simulink model "Simscape_CAD_Raibert"  (R2022a)
settings: Solver=VariableStepAuto  StartTime=0.0  StopTime=6  FixedStep=1E-6  MaxStep=1E-5  RelTol=1E-9
undefined symbols (not defined in the file or in its folder): arm_l, arm_r, arm_spacing, base_h, base_r, contactTime, desired_speed, height_plane, hip_bend_factor, hip_fuzz, initHip, initKnee, k_landing_angle, knee_bend_factor, knee_fuzz, lower_leg_length, max_torque, plane_x, plane_y, plane_z, upper_leg_length, X, Y, Z
libraries: sm_lib x46, nesl_utility x14, slpidlib x6, simulink x1
(part 1 of 3)
settings Model: SimulationMode=accelerator  Creator=Bradley Kwan  LastModifiedBy=jack3
settings SolverCC: ZeroCrossAlgorithm=Adaptive  AlgebraicLoopSolver=TrustRegion
settings DebuggingCC: UnconnectedInputMsg=warning  UnconnectedOutputMsg=warning  UnconnectedLineMsg=warning  SFMachineParentedDataDiag=warning
settings RTWCC: DLArmComputeVersion=19.05
settings ExplorerConfigSet: InternalSimMechanicsExplorerSettings="<ExplorerConfiguration><canonicalview>default</canonicalview><AnimationSetting><BasePlaybackSpeed>1.0</BasePlaybackSpeed><PlaybackSpeedFactor>1.0</PlaybackSpeedFactor></AnimationSetting><TilePanel><TileInfo><Tiles Columns=\"1\" Count=\"1\" Rows=\"1\"><Column Weight=\"1\"/><Row Weight=\"1\"/><Tile Height=\"1\" Width=\"1\" X=\"0\" Y=\"0\"/></Tiles></TileInfo><SceneInfo><SceneViewer><BGColor><R>0.60000002384185791</R><G>0.60000002384185791</G><B>0.60000002384185791</B></BGColor><Camera><DoPerspective>off</DoPerspective><Position><X>1.00328009491088266</X><Y>0.290256330840329813</Y><Z>0.225430262208942023</Z></Position><Center><X>0.0386568878869436583</X><Y>0.0720479721949161545</Y><Z>0.0774870951204086611</Z></Center><Up><X>-0.177845876958520221</X><Y>0.124361864790182741</Y><Z>0.976168515490416722</Z></Up><ViewLimDist>1</ViewLimDist><YLim>0.220252111002240375</YLim><XLim>0.209173030971946589</XLim></Camera></SceneViewer></SceneInfo></TilePanel><MechEditorPanel><Cameras/><GfxPanelCameraMap/><VideoCreator><PlaybackSpeedRatio>1.0</PlaybackSpeedRatio><FrameRate>60</FrameRate><VideoFormat>MPEG-4</VideoFormat><FrameSize>auto</FrameSize></VideoCreator></MechEditorPanel></ExplorerConfiguration>"

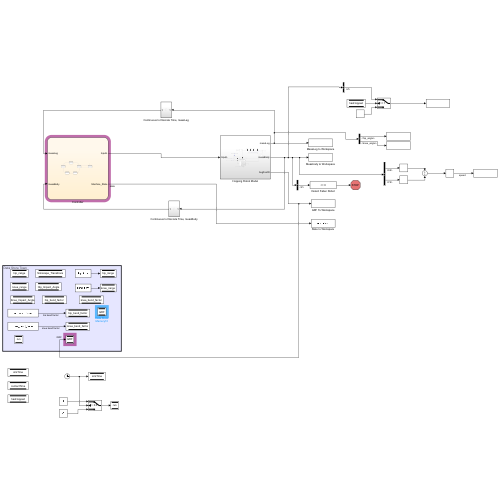
[thumbnail: Simulink's stored preview of the top-level diagram]
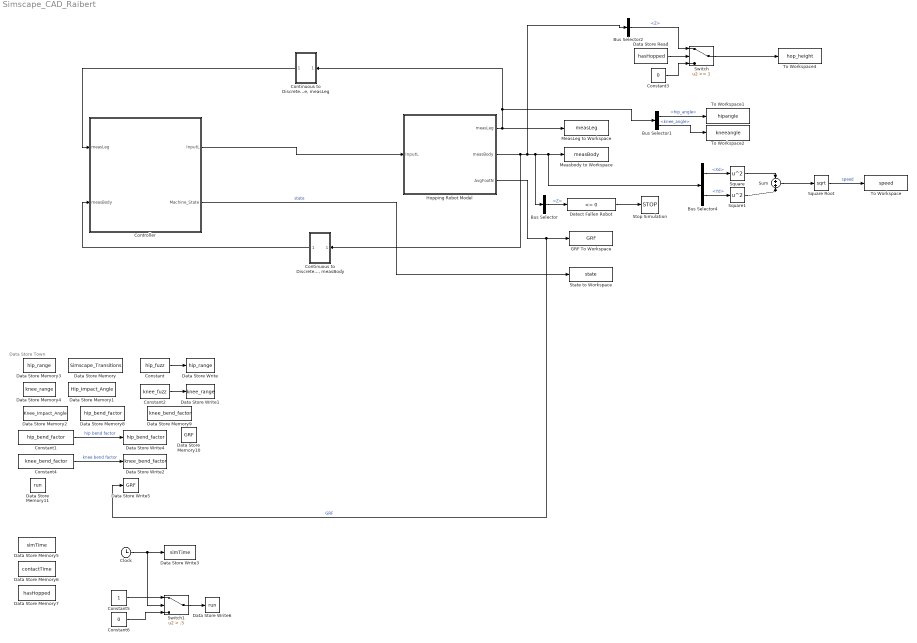
== system Simscape_CAD_Raibert ==
  note: Data Store Town
  Bus Selector : BusSelector  OutputSignals=Z
  Bus Selector1 : BusSelector  OutputSignals=hip_angle,knee_angle
  Bus Selector2 : BusSelector  OutputSignals=Z
  Bus Selector4 : BusSelector  OutputSignals=Xd,Yd
  Clock : Clock
  Constant : Constant  Value=hip_fuzz
  Constant1 : Constant  Value=hip_bend_factor
  Constant2 : Constant  Value=knee_fuzz
  Constant3 : Constant  Value=0
  Constant4 : Constant  Value=knee_bend_factor
  Constant5 : Constant
  Constant6 : Constant  Value=0
  "Continuous to Discrete Time, measBody" : Subsystem
  "Continuous to Discrete Time, measLeg" : Subsystem
  Controller : Stateflow chart  TreatAsAtomicUnit=on
  Data Store Memory : DataStoreMemory  DataStoreName=Simscape_Transitions  WriteAfterWriteMsg=warning  ShowAdditionalParam=off  OutDataTypeStr=double  Dimensions=3
  Data Store Memory1 : DataStoreMemory  DataStoreName=Hip_Impact_Angle  WriteAfterWriteMsg=warning  ShowAdditionalParam=off  OutDataTypeStr=double
  Data Store Memory10 : DataStoreMemory  DataStoreName=GRF  WriteAfterWriteMsg=warning  ShowAdditionalParam=off  OutDataTypeStr=double
  Data Store Memory11 : DataStoreMemory  DataStoreName=run  WriteAfterWriteMsg=warning  ShowAdditionalParam=off  OutDataTypeStr=double
  Data Store Memory2 : DataStoreMemory  DataStoreName=Knee_Impact_Angle  WriteAfterWriteMsg=warning  ShowAdditionalParam=off  OutDataTypeStr=double
  Data Store Memory3 : DataStoreMemory  DataStoreName=hip_range  WriteAfterWriteMsg=warning  ShowAdditionalParam=off  OutDataTypeStr=double
  Data Store Memory4 : DataStoreMemory  DataStoreName=knee_range  WriteAfterWriteMsg=warning  ShowAdditionalParam=off  OutDataTypeStr=double
  Data Store Memory5 : DataStoreMemory  DataStoreName=simTime  WriteAfterWriteMsg=warning  ShowAdditionalParam=off  OutDataTypeStr=double
  Data Store Memory6 : DataStoreMemory  DataStoreName=contactTime  WriteAfterWriteMsg=warning  ShowAdditionalParam=off  OutDataTypeStr=double
  Data Store Memory7 : DataStoreMemory  DataStoreName=hasHopped  WriteAfterWriteMsg=warning  ShowAdditionalParam=off  OutDataTypeStr=double
  Data Store Memory8 : DataStoreMemory  DataStoreName=hip_bend_factor  WriteAfterWriteMsg=warning  ShowAdditionalParam=off  OutDataTypeStr=double
  Data Store Memory9 : DataStoreMemory  DataStoreName=knee_bend_factor  WriteAfterWriteMsg=warning  ShowAdditionalParam=off  OutDataTypeStr=double
  Data Store Read : DataStoreRead  DataStoreName=hasHopped  IndexOptions=Index vector (dialog)  Indices=1  OutputSizes=1
  Data Store Write : DataStoreWrite  DataStoreName=hip_range  IndexOptions=Index vector (dialog)  Indices=1  OutputSizes=1
  Data Store Write1 : DataStoreWrite  DataStoreName=knee_range  IndexOptions=Index vector (dialog)  Indices=1  OutputSizes=1
  Data Store Write2 : DataStoreWrite  DataStoreName=knee_bend_factor  IndexOptions=Index vector (dialog)  Indices=1  OutputSizes=1
  Data Store Write3 : DataStoreWrite  DataStoreName=simTime  IndexOptions=Index vector (dialog)  Indices=1  OutputSizes=1
  Data Store Write4 : DataStoreWrite  DataStoreName=hip_bend_factor  IndexOptions=Index vector (dialog)  Indices=1  OutputSizes=1
  Data Store Write5 : DataStoreWrite  DataStoreName=GRF  IndexOptions=Index vector (dialog)  Indices=1  OutputSizes=1
  Data Store Write6 : DataStoreWrite  DataStoreName=run  IndexOptions=Index vector (dialog)  Indices=1  OutputSizes=1
  Detect Fallen Robot : simulink/Logic and Bit Operations/Compare To Constant  relop=<=  const=0  OutDataTypeStr=boolean
  GRF To Workspace : ToWorkspace  VariableName=GRF  SampleTime=-1
  Hopping Robot Model : Subsystem
  MeasLeg to Workspace : ToWorkspace  VariableName=measLeg  SampleTime=-1
  Measbody to Workspace : ToWorkspace  VariableName=measBody  SampleTime=-1
  Square : Math  Operator=square
  Square Root : Sqrt
  Square1 : Math  Operator=square
  State to Workspace : ToWorkspace  VariableName=state  SampleTime=-1
  Stop Simulation : Stop
  Sum : Sum  Inputs=+|+
  Switch : Switch  Threshold=1  SaturateOnIntegerOverflow=off  InputSameDT=off
  Switch1 : Switch  Criteria=u2 > Threshold  Threshold=.5  SaturateOnIntegerOverflow=off  InputSameDT=off
  To Workspace : ToWorkspace  VariableName=speed  SaveFormat=Timeseries  SampleTime=-1
  To Workspace1 : ToWorkspace  VariableName=hipangle  SaveFormat=Timeseries  SampleTime=-1
  To Workspace2 : ToWorkspace  VariableName=kneeangle  SaveFormat=Timeseries  SampleTime=-1
  To Workspace4 : ToWorkspace  VariableName=hop_height  SaveFormat=Timeseries  SampleTime=-1
  wires:
  Hopping Robot Model/2(measBody) -> "Continuous to Discrete Time, measBody"/1(In1), Bus Selector2/1, Bus Selector/1, Bus Selector4/1, Measbody to Workspace/1
  Bus Selector/1 -> Detect Fallen Robot/1  "<Z>"
  Detect Fallen Robot/1 -> Stop Simulation/1
  Hopping Robot Model/3(AvgFootN) -> Data Store Write5/1, GRF To Workspace/1  "GRF"
  Controller/1(InputL) -> Hopping Robot Model/1(InputL)
  Constant1/1 -> Data Store Write4/1  "hip bend factor"
  Controller/2(Machine_State) -> State to Workspace/1  "state"
  Constant4/1 -> Data Store Write2/1  "knee bend factor"
  Constant/1 -> Data Store Write/1
  Constant2/1 -> Data Store Write1/1
  Bus Selector4/2 -> Square1/1  "<Yd>"
  Bus Selector4/1 -> Square/1  "<Xd>"
  Square/1 -> Sum/1
  Square1/1 -> Sum/2
  Sum/1 -> Square Root/1
  Square Root/1 -> To Workspace/1  "speed"
  "Continuous to Discrete Time, measBody"/1(Out1) -> Controller/2(measBody)
  "Continuous to Discrete Time, measLeg"/1(Out1) -> Controller/1(measLeg)
  Bus Selector1/1 -> To Workspace1/1  "<hip_angle>"
  Bus Selector1/2 -> To Workspace2/1  "<knee_angle>"
  Data Store Read/1 -> Switch/2
  Switch/1 -> To Workspace4/1
  Hopping Robot Model/1(measLeg) -> Bus Selector1/1, "Continuous to Discrete Time, measLeg"/1(In1), MeasLeg to Workspace/1
  Constant3/1 -> Switch/3
  Bus Selector2/1 -> Switch/1  "<Z>"
  Switch1/1 -> Data Store Write6/1
  Constant6/1 -> Switch1/3
  Constant5/1 -> Switch1/1
  Clock/1 -> Switch1/2, Data Store Write3/1

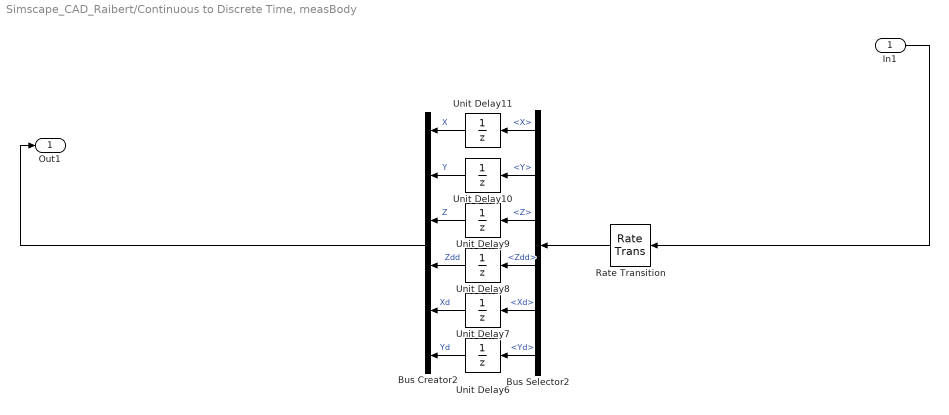
== system Simscape_CAD_Raibert/Continuous to Discrete Time, measBody ==
  In1 : Inport
  Bus Creator2 : BusCreator  Inputs=6
  Bus Selector2 : BusSelector  OutputSignals=X,Y,Z,Zdd,Xd,Yd
  Rate Transition : RateTransition
  Unit Delay{6..11} (6 alike) : UnitDelay  SampleTime=-1  HasFrameUpgradeWarning=on
  Out1 : Outport
  wires:
  Unit Delay7/1 -> Bus Creator2/5  "Xd"
  Bus Selector2/1 -> Unit Delay11/1  "<X>"
  Bus Selector2/6 -> Unit Delay6/1  "<Yd>"
  Bus Selector2/3 -> Unit Delay9/1  "<Z>"
  Bus Selector2/2 -> Unit Delay10/1  "<Y>"
  Bus Selector2/5 -> Unit Delay7/1  "<Xd>"
  Bus Selector2/4 -> Unit Delay8/1  "<Zdd>"
  Unit Delay8/1 -> Bus Creator2/4  "Zdd"
  Rate Transition/1 -> Bus Selector2/1
  Unit Delay10/1 -> Bus Creator2/2  "Y"
  Unit Delay11/1 -> Bus Creator2/1  "X"
  Unit Delay9/1 -> Bus Creator2/3  "Z"
  Unit Delay6/1 -> Bus Creator2/6  "Yd"
  In1/1 -> Rate Transition/1
  Bus Creator2/1 -> Out1/1

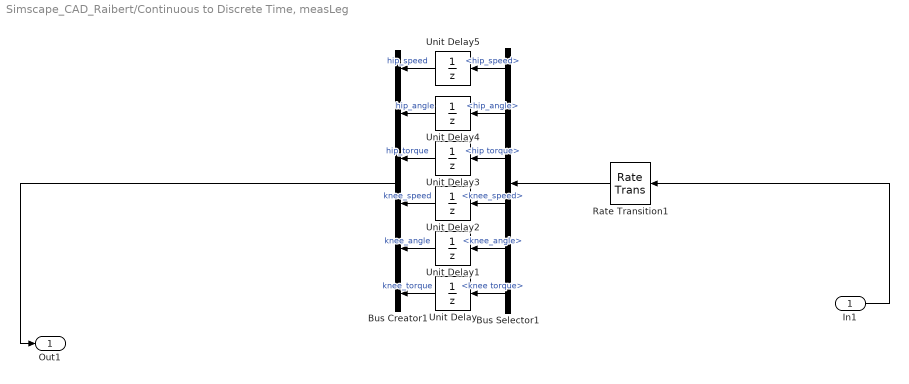
== system Simscape_CAD_Raibert/Continuous to Discrete Time, measLeg ==
  In1 : Inport
  Bus Creator1 : BusCreator  Inputs=6
  Bus Selector1 : BusSelector  OutputSignals=hip_speed,hip_angle,hip torque,knee_speed,knee_angle,knee torque
  Rate Transition1 : RateTransition
  Unit Delay{,1..5} (6 alike) : UnitDelay  SampleTime=-1  HasFrameUpgradeWarning=on
  Out1 : Outport
  wires:
  Bus Selector1/1 -> Unit Delay5/1  "<hip_speed>"
  Bus Selector1/6 -> Unit Delay/1  "<knee torque>"
  Unit Delay4/1 -> Bus Creator1/2  "hip_angle"
  Rate Transition1/1 -> Bus Selector1/1
  Bus Selector1/4 -> Unit Delay2/1  "<knee_speed>"
  Unit Delay2/1 -> Bus Creator1/4  "knee_speed"
  Unit Delay1/1 -> Bus Creator1/5  "knee_angle"
  Bus Creator1/1 -> Out1/1
  Unit Delay5/1 -> Bus Creator1/1  "hip_speed"
  Bus Selector1/5 -> Unit Delay1/1  "<knee_angle>"
  Bus Selector1/3 -> Unit Delay3/1  "<hip torque>"
  Unit Delay/1 -> Bus Creator1/6  "knee_torque"
  Unit Delay3/1 -> Bus Creator1/3  "hip_torque"
  Bus Selector1/2 -> Unit Delay4/1  "<hip_angle>"
  In1/1 -> Rate Transition1/1

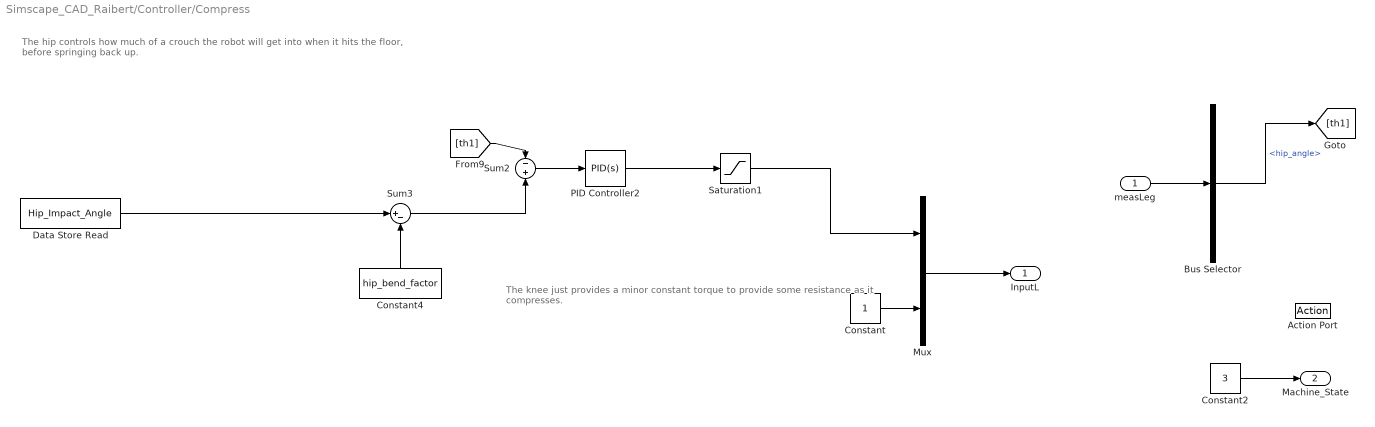
== system Simscape_CAD_Raibert/Controller/Compress ==
  note: The knee just provides a minor constant torque to provide some resistance
      | as it compresses.
  note: The hip controls how much of a crouch the robot will get into when it hits the floor,
      | before springing back up.
  measLeg : Inport
  Action Port : ActionPort
      settings: CopyFcn=Stateflow.SLINSF.SimulinkMan.removeBlockPreDeleteFcn  PreDeleteFcn=Stateflow.SLINSF.SimulinkMan.unsafePredeleteFcn
  Bus Selector : BusSelector  OutputSignals=hip_angle
  Constant : Constant
  Constant2 : Constant  Value=3
  Constant4 : Constant  Value=hip_bend_factor
  Data Store Read : DataStoreRead  DataStoreName=Hip_Impact_Angle  IndexOptions=Index vector (dialog)  Indices=1  OutputSizes=1
  Mux : Mux  Inputs=2
  PID Controller2 : slpidlib/PID Controller  Controller=PID  Form=Parallel  TimeDomain=Continuous-time  UseExternalTs=off  SampleTime=-1  IntegratorMethod=Forward Euler  FilterMethod=Forward Euler  ControllerParametersSource=internal  P=100  I=0  UseKiTs=off  D=10  N=100  UseFilter=on  TunerSelectOption=Transfer Function Based (PID Tuner App)  InitialConditionSource=internal  InitialConditionForIntegrator=0  InitialConditionForFilter=0  DifferentiatorICPrevScaledInput=0  ExternalReset=none  TrackingMode=off  Kt=1  LimitOutput=off  SatLimitsSource=internal  UpperSaturationLimit=inf  LowerSaturationLimit=-inf  LinearizeAsGain=on  AntiWindupMode=none  Kb=1  POutMin=[]  POutMax=[]  IOutMin=[]  IOutMax=[]  DOutMin=[]  DOutMax=[]  NOutMin=[]  NOutMax=[]  SumOutMin=[]  SumOutMax=[]  SaturationOutMin=[]  SaturationOutMax=[]  PParamMin=[]  PParamMax=[]  IParamMin=[]  IParamMax=[]  DParamMin=[]  DParamMax=[]  NParamMin=[]  NParamMax=[]  KbParamMin=[]  KbParamMax=[]  KtParamMin=[]  KtParamMax=[]  KbOutMin=[]  KbOutMax=[]  KtOutMin=[]  KtOutMax=[]  IntegratorOutMin=[]  IntegratorOutMax=[]  FilterOutMin=[]  FilterOutMax=[]  SumI1OutMin=[]  SumI1OutMax=[]  SumI2OutMin=[]  SumI2OutMax=[]  SumI3OutMin=[]  SumI3OutMax=[]  SumI4OutMin=[]  SumI4OutMax=[]  SumDOutMin=[]  SumDOutMax=[]  DifferentiatorOutMin=[]  DifferentiatorOutMax=[]  FilterDiffOutCoefMin=[]  FilterDiffOutCoefMax=[]  ReciprocalOutMin=[]  ReciprocalOutMax=[]  SumDenOutMin=[]  SumDenOutMax=[]  SumNumOutMin=[]  SumNumOutMax=[]  DivideOutMin=[]  DivideOutMax=[]  UdiffTsProdOutMin=[]  UdiffTsProdOutMax=[]  NTsProdOutMin=[]  NTsProdOutMax=[]  UintegralTsProdOutMin=[]  UintegralTsProdOutMax=[]  UngainTsProdOutMin=[]  UngainTsProdOutMax=[]  IntegratorContinuousStateAttributes=''  IntegratorStateMustResolveToSignalObject=off  IntegratorRTWStateStorageClass=Auto  FilterContinuousStateAttributes=''  FilterStateMustResolveToSignalObject=off  FilterRTWStateStorageClass=Auto  ParallelPVariant=InternalParameters  IdealPVariant=Disabled  IVariant=InternalParameters  DVariant=InternalParameters  IntegratorVariant=Continuous  SatVariant=Disabled  AWVariant=Passthrough  PCopyVariant=Disabled  TRVariant=Disabled  FdbkBlocksVariant=Forward  IdealPFdbkVariant=Disabled  SatFdbkVariant=Disabled  DerivativeFilterVariant=ContFilter  NVariant=InternalParameters  NCopyVariant=Disabled  FilterICVariant=InternalICsFilter  IntegratorICVariant=InternalICs  ExternalResetVariant=Disabled  TRSumVariant=Passthrough  SumFdbkVariant=Disabled  SumVariant=Sum_PID  TsampFilterVariant=InternalTs  TsampNgainVariant=Passthrough  TsampIntegralVariant=Passthrough  ExternalSaturationOutDataTypeStr=Inherit: Same as second input  aMode=0
  Saturation1 : Saturate  UpperLimit=8  LowerLimit=-8
  Sum2 : Sum  Inputs=-+
  Sum3 : Sum  Inputs=|+-
  InputL : Outport
  Machine_State : Outport  Port=2
  wires:
  measLeg/1 -> Bus Selector/1
  Bus Selector/1 -> [th1]  "<hip_angle>"
  Mux/1 -> InputL/1
  Constant2/1 -> Machine_State/1
  PID Controller2/1 -> Saturation1/1
  [th1] -> Sum2/1
  Data Store Read/1 -> Sum3/1
  Saturation1/1 -> Mux/1
  Constant4/1 -> Sum3/2
  Sum3/1 -> Sum2/2
  Sum2/1 -> PID Controller2/1
  Constant/1 -> Mux/2

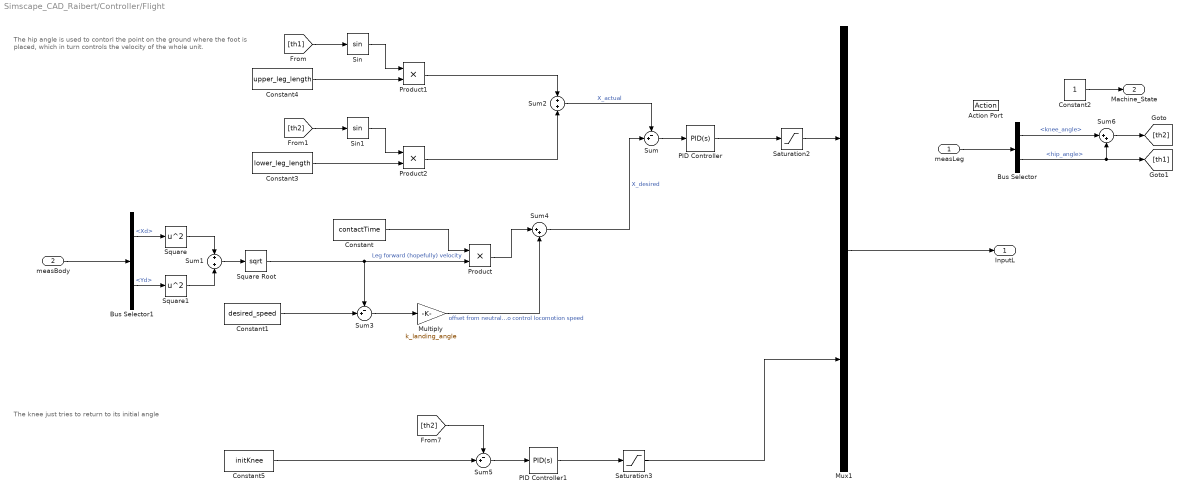
== system Simscape_CAD_Raibert/Controller/Flight ==
  note: The knee just tries to return to its initial angle
  note: The hip angle is used to contorl the point on the ground where the foot is
      | placed, which in turn controls the velocity of the whole unit.
  measLeg : Inport
  measBody : Inport  Port=2
  Action Port : ActionPort
      settings: CopyFcn=Stateflow.SLINSF.SimulinkMan.removeBlockPreDeleteFcn  PreDeleteFcn=Stateflow.SLINSF.SimulinkMan.unsafePredeleteFcn
  Bus Selector : BusSelector  OutputSignals=knee_angle,hip_angle
  Bus Selector1 : BusSelector  OutputSignals=Xd,Yd
  Constant : Constant  Value=contactTime
  Constant1 : Constant  Value=desired_speed  SampleTime=-1
  Constant2 : Constant
  Constant3 : Constant  Value=lower_leg_length
  Constant4 : Constant  Value=upper_leg_length
  Constant5 : Constant  Value=initKnee
  Multiply : Gain  Gain=k_landing_angle
  Mux1 : Mux  Inputs=2
  PID Controller : slpidlib/PID Controller  Controller=PID  Form=Parallel  TimeDomain=Continuous-time  UseExternalTs=off  SampleTime=-1  IntegratorMethod=Forward Euler  FilterMethod=Forward Euler  ControllerParametersSource=internal  P=50  I=0  UseKiTs=off  D=10  N=100  UseFilter=on  TunerSelectOption=Transfer Function Based (PID Tuner App)  InitialConditionSource=internal  InitialConditionForIntegrator=0  InitialConditionForFilter=0  DifferentiatorICPrevScaledInput=0  ExternalReset=none  TrackingMode=off  Kt=1  LimitOutput=off  SatLimitsSource=internal  UpperSaturationLimit=inf  LowerSaturationLimit=-inf  LinearizeAsGain=on  AntiWindupMode=none  Kb=1  POutMin=[]  POutMax=[]  IOutMin=[]  IOutMax=[]  DOutMin=[]  DOutMax=[]  NOutMin=[]  NOutMax=[]  SumOutMin=[]  SumOutMax=[]  SaturationOutMin=[]  SaturationOutMax=[]  PParamMin=[]  PParamMax=[]  IParamMin=[]  IParamMax=[]  DParamMin=[]  DParamMax=[]  NParamMin=[]  NParamMax=[]  KbParamMin=[]  KbParamMax=[]  KtParamMin=[]  KtParamMax=[]  KbOutMin=[]  KbOutMax=[]  KtOutMin=[]  KtOutMax=[]  IntegratorOutMin=[]  IntegratorOutMax=[]  FilterOutMin=[]  FilterOutMax=[]  SumI1OutMin=[]  SumI1OutMax=[]  SumI2OutMin=[]  SumI2OutMax=[]  SumI3OutMin=[]  SumI3OutMax=[]  SumI4OutMin=[]  SumI4OutMax=[]  SumDOutMin=[]  SumDOutMax=[]  DifferentiatorOutMin=[]  DifferentiatorOutMax=[]  FilterDiffOutCoefMin=[]  FilterDiffOutCoefMax=[]  ReciprocalOutMin=[]  ReciprocalOutMax=[]  SumDenOutMin=[]  SumDenOutMax=[]  SumNumOutMin=[]  SumNumOutMax=[]  DivideOutMin=[]  DivideOutMax=[]  UdiffTsProdOutMin=[]  UdiffTsProdOutMax=[]  NTsProdOutMin=[]  NTsProdOutMax=[]  UintegralTsProdOutMin=[]  UintegralTsProdOutMax=[]  UngainTsProdOutMin=[]  UngainTsProdOutMax=[]  IntegratorContinuousStateAttributes=''  IntegratorStateMustResolveToSignalObject=off  IntegratorRTWStateStorageClass=Auto  FilterContinuousStateAttributes=''  FilterStateMustResolveToSignalObject=off  FilterRTWStateStorageClass=Auto  ParallelPVariant=InternalParameters  IdealPVariant=Disabled  IVariant=InternalParameters  DVariant=InternalParameters  IntegratorVariant=Continuous  SatVariant=Disabled  AWVariant=Passthrough  PCopyVariant=Disabled  TRVariant=Disabled  FdbkBlocksVariant=Forward  IdealPFdbkVariant=Disabled  SatFdbkVariant=Disabled  DerivativeFilterVariant=ContFilter  NVariant=InternalParameters  NCopyVariant=Disabled  FilterICVariant=InternalICsFilter  IntegratorICVariant=InternalICs  ExternalResetVariant=Disabled  TRSumVariant=Passthrough  SumFdbkVariant=Disabled  SumVariant=Sum_PID  TsampFilterVariant=InternalTs  TsampNgainVariant=Passthrough  TsampIntegralVariant=Passthrough  ExternalSaturationOutDataTypeStr=Inherit: Same as second input  aMode=0
  PID Controller1 : slpidlib/PID Controller  Controller=PID  Form=Parallel  TimeDomain=Continuous-time  UseExternalTs=off  SampleTime=-1  IntegratorMethod=Forward Euler  FilterMethod=Forward Euler  ControllerParametersSource=internal  P=50  I=0  UseKiTs=off  D=5  N=100  UseFilter=on  TunerSelectOption=Transfer Function Based (PID Tuner App)  InitialConditionSource=internal  InitialConditionForIntegrator=0  InitialConditionForFilter=0  DifferentiatorICPrevScaledInput=0  ExternalReset=none  TrackingMode=off  Kt=1  LimitOutput=off  SatLimitsSource=internal  UpperSaturationLimit=inf  LowerSaturationLimit=-inf  LinearizeAsGain=on  AntiWindupMode=none  Kb=1  POutMin=[]  POutMax=[]  IOutMin=[]  IOutMax=[]  DOutMin=[]  DOutMax=[]  NOutMin=[]  NOutMax=[]  SumOutMin=[]  SumOutMax=[]  SaturationOutMin=[]  SaturationOutMax=[]  PParamMin=[]  PParamMax=[]  IParamMin=[]  IParamMax=[]  DParamMin=[]  DParamMax=[]  NParamMin=[]  NParamMax=[]  KbParamMin=[]  KbParamMax=[]  KtParamMin=[]  KtParamMax=[]  KbOutMin=[]  KbOutMax=[]  KtOutMin=[]  KtOutMax=[]  IntegratorOutMin=[]  IntegratorOutMax=[]  FilterOutMin=[]  FilterOutMax=[]  SumI1OutMin=[]  SumI1OutMax=[]  SumI2OutMin=[]  SumI2OutMax=[]  SumI3OutMin=[]  SumI3OutMax=[]  SumI4OutMin=[]  SumI4OutMax=[]  SumDOutMin=[]  SumDOutMax=[]  DifferentiatorOutMin=[]  DifferentiatorOutMax=[]  FilterDiffOutCoefMin=[]  FilterDiffOutCoefMax=[]  ReciprocalOutMin=[]  ReciprocalOutMax=[]  SumDenOutMin=[]  SumDenOutMax=[]  SumNumOutMin=[]  SumNumOutMax=[]  DivideOutMin=[]  DivideOutMax=[]  UdiffTsProdOutMin=[]  UdiffTsProdOutMax=[]  NTsProdOutMin=[]  NTsProdOutMax=[]  UintegralTsProdOutMin=[]  UintegralTsProdOutMax=[]  UngainTsProdOutMin=[]  UngainTsProdOutMax=[]  IntegratorContinuousStateAttributes=''  IntegratorStateMustResolveToSignalObject=off  IntegratorRTWStateStorageClass=Auto  FilterContinuousStateAttributes=''  FilterStateMustResolveToSignalObject=off  FilterRTWStateStorageClass=Auto  ParallelPVariant=InternalParameters  IdealPVariant=Disabled  IVariant=InternalParameters  DVariant=InternalParameters  IntegratorVariant=Continuous  SatVariant=Disabled  AWVariant=Passthrough  PCopyVariant=Disabled  TRVariant=Disabled  FdbkBlocksVariant=Forward  IdealPFdbkVariant=Disabled  SatFdbkVariant=Disabled  DerivativeFilterVariant=ContFilter  NVariant=InternalParameters  NCopyVariant=Disabled  FilterICVariant=InternalICsFilter  IntegratorICVariant=InternalICs  ExternalResetVariant=Disabled  TRSumVariant=Passthrough  SumFdbkVariant=Disabled  SumVariant=Sum_PID  TsampFilterVariant=InternalTs  TsampNgainVariant=Passthrough  TsampIntegralVariant=Passthrough  ExternalSaturationOutDataTypeStr=Inherit: Same as second input  aMode=0
  Product : Product
  Product1 : Product
  Product2 : Product
  Saturation2 : Saturate  UpperLimit=max_torque  LowerLimit=-max_torque
  Saturation3 : Saturate  UpperLimit=max_torque  LowerLimit=-max_torque
  Sin : Trigonometry
  Sin1 : Trigonometry
  Square : Math  Operator=square
  Square Root : Sqrt
  Square1 : Math  Operator=square
  Sum : Sum  Inputs=-+|
  Sum1 : Sum  Inputs=+|+
  Sum2 : Sum  Inputs=+|+
  Sum3 : Sum  Inputs=-+|
  Sum4 : Sum  Inputs=|++
  Sum5 : Sum  Inputs=-+|
  Sum6 : Sum  Inputs=|++
  InputL : Outport
  Machine_State : Outport  Port=2
  wires:
  Multiply/1 -> Sum4/2  "offset from neutral point to control locomotion speed"
  Sum3/1 -> Multiply/1
  Square Root/1 -> Product/2, Sum3/1  "Leg forward (hopefully) velocity"
  Sum4/1 -> Sum/2  "X_desired"
  Sum1/1 -> Square Root/1
  Bus Selector1/2 -> Square1/1  "<Yd>"
  Bus Selector1/1 -> Square/1  "<Xd>"
  Square/1 -> Sum1/1
  Square1/1 -> Sum1/2
  Constant1/1 -> Sum3/2
  PID Controller/1 -> Saturation2/1
  Constant5/1 -> Sum5/2
  PID Controller1/1 -> Saturation3/1
  Saturation3/1 -> Mux1/2
  Saturation2/1 -> Mux1/1
  Sum5/1 -> PID Controller1/1
  [th2] -> Sum5/1
  Mux1/1 -> InputL/1
  Bus Selector/1 -> Sum6/1  "<knee_angle>"
  measLeg/1 -> Bus Selector/1
  Constant/1 -> Product/1
  measBody/1 -> Bus Selector1/1
  Constant2/1 -> Machine_State/1
  Product/1 -> Sum4/1
  Sum/1 -> PID Controller/1
  Bus Selector/2 -> [th1], Sum6/2  "<hip_angle>"
  [th1] -> Sin/1
  Sin/1 -> Product1/1
  Constant4/1 -> Product1/2
  [th2] -> Sin1/1
  Constant3/1 -> Product2/2
  Sin1/1 -> Product2/1
  Sum2/1 -> Sum/1  "X_actual"
  Product1/1 -> Sum2/1
  Product2/1 -> Sum2/2
  Sum6/1 -> [th2]

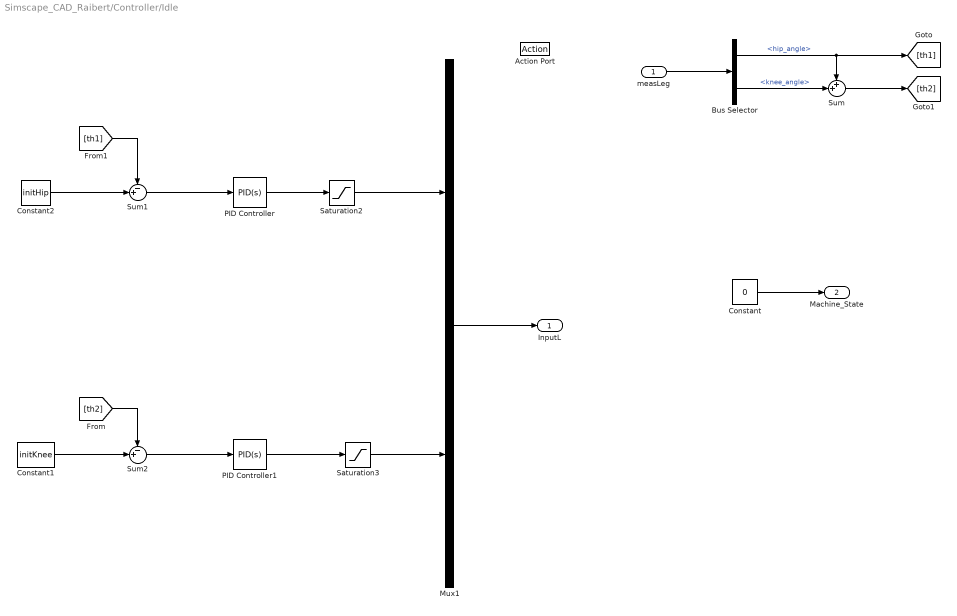
== system Simscape_CAD_Raibert/Controller/Idle ==
  measLeg : Inport
  Action Port : ActionPort
      settings: CopyFcn=Stateflow.SLINSF.SimulinkMan.removeBlockPreDeleteFcn  PreDeleteFcn=Stateflow.SLINSF.SimulinkMan.unsafePredeleteFcn
  Bus Selector : BusSelector  OutputSignals=hip_angle,knee_angle
  Constant : Constant  Value=0
  Constant1 : Constant  Value=initKnee
  Constant2 : Constant  Value=initHip
  Mux1 : Mux  Inputs=2
  PID Controller : slpidlib/PID Controller  Controller=PID  Form=Parallel  TimeDomain=Continuous-time  UseExternalTs=off  SampleTime=-1  IntegratorMethod=Forward Euler  FilterMethod=Forward Euler  ControllerParametersSource=internal  P=50  I=0  UseKiTs=off  D=10  N=100  UseFilter=on  TunerSelectOption=Transfer Function Based (PID Tuner App)  InitialConditionSource=internal  InitialConditionForIntegrator=0  InitialConditionForFilter=0  DifferentiatorICPrevScaledInput=0  ExternalReset=none  TrackingMode=off  Kt=1  LimitOutput=off  SatLimitsSource=internal  UpperSaturationLimit=inf  LowerSaturationLimit=-inf  LinearizeAsGain=on  AntiWindupMode=none  Kb=1  POutMin=[]  POutMax=[]  IOutMin=[]  IOutMax=[]  DOutMin=[]  DOutMax=[]  NOutMin=[]  NOutMax=[]  SumOutMin=[]  SumOutMax=[]  SaturationOutMin=[]  SaturationOutMax=[]  PParamMin=[]  PParamMax=[]  IParamMin=[]  IParamMax=[]  DParamMin=[]  DParamMax=[]  NParamMin=[]  NParamMax=[]  KbParamMin=[]  KbParamMax=[]  KtParamMin=[]  KtParamMax=[]  KbOutMin=[]  KbOutMax=[]  KtOutMin=[]  KtOutMax=[]  IntegratorOutMin=[]  IntegratorOutMax=[]  FilterOutMin=[]  FilterOutMax=[]  SumI1OutMin=[]  SumI1OutMax=[]  SumI2OutMin=[]  SumI2OutMax=[]  SumI3OutMin=[]  SumI3OutMax=[]  SumI4OutMin=[]  SumI4OutMax=[]  SumDOutMin=[]  SumDOutMax=[]  DifferentiatorOutMin=[]  DifferentiatorOutMax=[]  FilterDiffOutCoefMin=[]  FilterDiffOutCoefMax=[]  ReciprocalOutMin=[]  ReciprocalOutMax=[]  SumDenOutMin=[]  SumDenOutMax=[]  SumNumOutMin=[]  SumNumOutMax=[]  DivideOutMin=[]  DivideOutMax=[]  UdiffTsProdOutMin=[]  UdiffTsProdOutMax=[]  NTsProdOutMin=[]  NTsProdOutMax=[]  UintegralTsProdOutMin=[]  UintegralTsProdOutMax=[]  UngainTsProdOutMin=[]  UngainTsProdOutMax=[]  IntegratorContinuousStateAttributes=''  IntegratorStateMustResolveToSignalObject=off  IntegratorRTWStateStorageClass=Auto  FilterContinuousStateAttributes=''  FilterStateMustResolveToSignalObject=off  FilterRTWStateStorageClass=Auto  ParallelPVariant=InternalParameters  IdealPVariant=Disabled  IVariant=InternalParameters  DVariant=InternalParameters  IntegratorVariant=Continuous  SatVariant=Disabled  AWVariant=Passthrough  PCopyVariant=Disabled  TRVariant=Disabled  FdbkBlocksVariant=Forward  IdealPFdbkVariant=Disabled  SatFdbkVariant=Disabled  DerivativeFilterVariant=ContFilter  NVariant=InternalParameters  NCopyVariant=Disabled  FilterICVariant=InternalICsFilter  IntegratorICVariant=InternalICs  ExternalResetVariant=Disabled  TRSumVariant=Passthrough  SumFdbkVariant=Disabled  SumVariant=Sum_PID  TsampFilterVariant=InternalTs  TsampNgainVariant=Passthrough  TsampIntegralVariant=Passthrough  ExternalSaturationOutDataTypeStr=Inherit: Same as second input  aMode=0
  PID Controller1 : slpidlib/PID Controller  Controller=PID  Form=Parallel  TimeDomain=Continuous-time  UseExternalTs=off  SampleTime=-1  IntegratorMethod=Forward Euler  FilterMethod=Forward Euler  ControllerParametersSource=internal  P=50  I=0  UseKiTs=off  D=5  N=100  UseFilter=on  TunerSelectOption=Transfer Function Based (PID Tuner App)  InitialConditionSource=internal  InitialConditionForIntegrator=0  InitialConditionForFilter=0  DifferentiatorICPrevScaledInput=0  ExternalReset=none  TrackingMode=off  Kt=1  LimitOutput=off  SatLimitsSource=internal  UpperSaturationLimit=inf  LowerSaturationLimit=-inf  LinearizeAsGain=on  AntiWindupMode=none  Kb=1  POutMin=[]  POutMax=[]  IOutMin=[]  IOutMax=[]  DOutMin=[]  DOutMax=[]  NOutMin=[]  NOutMax=[]  SumOutMin=[]  SumOutMax=[]  SaturationOutMin=[]  SaturationOutMax=[]  PParamMin=[]  PParamMax=[]  IParamMin=[]  IParamMax=[]  DParamMin=[]  DParamMax=[]  NParamMin=[]  NParamMax=[]  KbParamMin=[]  KbParamMax=[]  KtParamMin=[]  KtParamMax=[]  KbOutMin=[]  KbOutMax=[]  KtOutMin=[]  KtOutMax=[]  IntegratorOutMin=[]  IntegratorOutMax=[]  FilterOutMin=[]  FilterOutMax=[]  SumI1OutMin=[]  SumI1OutMax=[]  SumI2OutMin=[]  SumI2OutMax=[]  SumI3OutMin=[]  SumI3OutMax=[]  SumI4OutMin=[]  SumI4OutMax=[]  SumDOutMin=[]  SumDOutMax=[]  DifferentiatorOutMin=[]  DifferentiatorOutMax=[]  FilterDiffOutCoefMin=[]  FilterDiffOutCoefMax=[]  ReciprocalOutMin=[]  ReciprocalOutMax=[]  SumDenOutMin=[]  SumDenOutMax=[]  SumNumOutMin=[]  SumNumOutMax=[]  DivideOutMin=[]  DivideOutMax=[]  UdiffTsProdOutMin=[]  UdiffTsProdOutMax=[]  NTsProdOutMin=[]  NTsProdOutMax=[]  UintegralTsProdOutMin=[]  UintegralTsProdOutMax=[]  UngainTsProdOutMin=[]  UngainTsProdOutMax=[]  IntegratorContinuousStateAttributes=''  IntegratorStateMustResolveToSignalObject=off  IntegratorRTWStateStorageClass=Auto  FilterContinuousStateAttributes=''  FilterStateMustResolveToSignalObject=off  FilterRTWStateStorageClass=Auto  ParallelPVariant=InternalParameters  IdealPVariant=Disabled  IVariant=InternalParameters  DVariant=InternalParameters  IntegratorVariant=Continuous  SatVariant=Disabled  AWVariant=Passthrough  PCopyVariant=Disabled  TRVariant=Disabled  FdbkBlocksVariant=Forward  IdealPFdbkVariant=Disabled  SatFdbkVariant=Disabled  DerivativeFilterVariant=ContFilter  NVariant=InternalParameters  NCopyVariant=Disabled  FilterICVariant=InternalICsFilter  IntegratorICVariant=InternalICs  ExternalResetVariant=Disabled  TRSumVariant=Passthrough  SumFdbkVariant=Disabled  SumVariant=Sum_PID  TsampFilterVariant=InternalTs  TsampNgainVariant=Passthrough  TsampIntegralVariant=Passthrough  ExternalSaturationOutDataTypeStr=Inherit: Same as second input  aMode=0
  Saturation2 : Saturate  UpperLimit=max_torque  LowerLimit=-max_torque
  Saturation3 : Saturate  UpperLimit=max_torque  LowerLimit=-max_torque
  Sum : Sum  Inputs=++|
  Sum1 : Sum  Inputs=-+|
  Sum2 : Sum  Inputs=-+|
  InputL : Outport
  Machine_State : Outport  Port=2
  wires:
  PID Controller/1 -> Saturation2/1
  Saturation3/1 -> Mux1/2
  Saturation2/1 -> Mux1/1
  Mux1/1 -> InputL/1
  PID Controller1/1 -> Saturation3/1
  Constant/1 -> Machine_State/1
  measLeg/1 -> Bus Selector/1
  Bus Selector/2 -> Sum/2  "<knee_angle>"
  Bus Selector/1 -> Sum/1, [th1]  "<hip_angle>"
  Sum/1 -> [th2]
  Sum1/1 -> PID Controller/1
  Sum2/1 -> PID Controller1/1
  [th2] -> Sum2/1
  Constant1/1 -> Sum2/2
  [th1] -> Sum1/1
  Constant2/1 -> Sum1/2

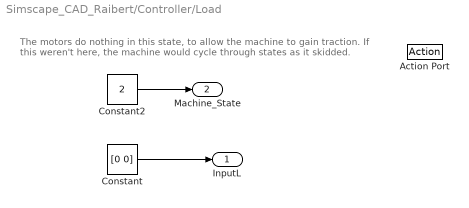
== system Simscape_CAD_Raibert/Controller/Load ==
  note: The motors do nothing in this state, to allow the machine to gain traction.
      | If this weren't here, the machine would cycle through states as it skidded.
  Action Port : ActionPort
      settings: CopyFcn=Stateflow.SLINSF.SimulinkMan.removeBlockPreDeleteFcn  PreDeleteFcn=Stateflow.SLINSF.SimulinkMan.unsafePredeleteFcn
  Constant : Constant  Value=[0 0]  VectorParams1D=off
  Constant2 : Constant  Value=2
  InputL : Outport
  Machine_State : Outport  Port=2
  wires:
  Constant/1 -> InputL/1
  Constant2/1 -> Machine_State/1

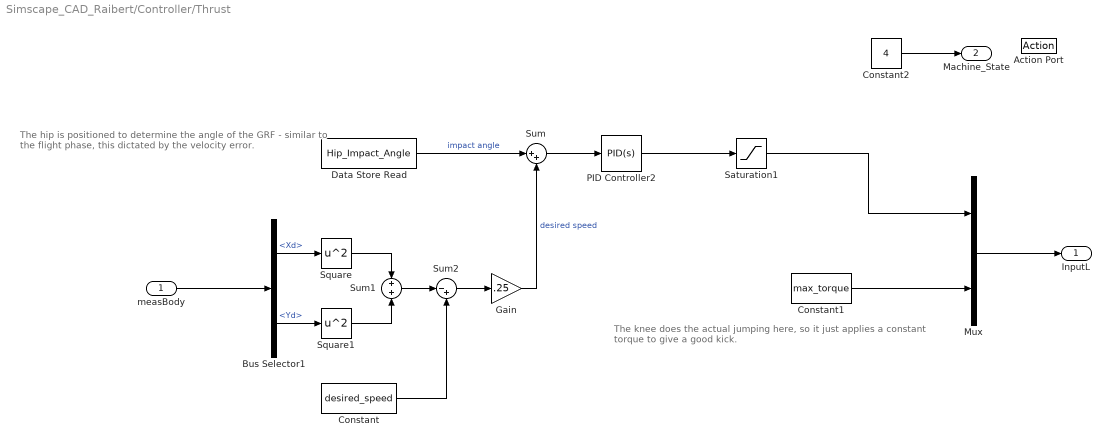
== system Simscape_CAD_Raibert/Controller/Thrust ==
  note: The knee does the actual jumping here, so it just applies a constant
      | torque to give a good kick.
  note: The hip is positioned to determine the angle of the GRF - similar
      | to the flight phase, this dictated by the velocity error.
  measBody : Inport
  Action Port : ActionPort
      settings: CopyFcn=Stateflow.SLINSF.SimulinkMan.removeBlockPreDeleteFcn  PreDeleteFcn=Stateflow.SLINSF.SimulinkMan.unsafePredeleteFcn
  Bus Selector1 : BusSelector  OutputSignals=Xd,Yd
  Constant : Constant  Value=desired_speed
  Constant1 : Constant  Value=max_torque
  Constant2 : Constant  Value=4
  Data Store Read : DataStoreRead  DataStoreName=Hip_Impact_Angle  IndexOptions=Index vector (dialog)  Indices=1  OutputSizes=1
  Gain : Gain  Gain=.25
  Mux : Mux  Inputs=2
  PID Controller2 : slpidlib/PID Controller  Controller=PID  Form=Parallel  TimeDomain=Continuous-time  UseExternalTs=off  SampleTime=-1  IntegratorMethod=Forward Euler  FilterMethod=Forward Euler  ControllerParametersSource=internal  P=50  I=0  UseKiTs=off  D=10  N=100  UseFilter=on  TunerSelectOption=Transfer Function Based (PID Tuner App)  InitialConditionSource=internal  InitialConditionForIntegrator=0  InitialConditionForFilter=0  DifferentiatorICPrevScaledInput=0  ExternalReset=none  TrackingMode=off  Kt=1  LimitOutput=off  SatLimitsSource=internal  UpperSaturationLimit=inf  LowerSaturationLimit=-inf  LinearizeAsGain=on  AntiWindupMode=none  Kb=1  POutMin=[]  POutMax=[]  IOutMin=[]  IOutMax=[]  DOutMin=[]  DOutMax=[]  NOutMin=[]  NOutMax=[]  SumOutMin=[]  SumOutMax=[]  SaturationOutMin=[]  SaturationOutMax=[]  PParamMin=[]  PParamMax=[]  IParamMin=[]  IParamMax=[]  DParamMin=[]  DParamMax=[]  NParamMin=[]  NParamMax=[]  KbParamMin=[]  KbParamMax=[]  KtParamMin=[]  KtParamMax=[]  KbOutMin=[]  KbOutMax=[]  KtOutMin=[]  KtOutMax=[]  IntegratorOutMin=[]  IntegratorOutMax=[]  FilterOutMin=[]  FilterOutMax=[]  SumI1OutMin=[]  SumI1OutMax=[]  SumI2OutMin=[]  SumI2OutMax=[]  SumI3OutMin=[]  SumI3OutMax=[]  SumI4OutMin=[]  SumI4OutMax=[]  SumDOutMin=[]  SumDOutMax=[]  DifferentiatorOutMin=[]  DifferentiatorOutMax=[]  FilterDiffOutCoefMin=[]  FilterDiffOutCoefMax=[]  ReciprocalOutMin=[]  ReciprocalOutMax=[]  SumDenOutMin=[]  SumDenOutMax=[]  SumNumOutMin=[]  SumNumOutMax=[]  DivideOutMin=[]  DivideOutMax=[]  UdiffTsProdOutMin=[]  UdiffTsProdOutMax=[]  NTsProdOutMin=[]  NTsProdOutMax=[]  UintegralTsProdOutMin=[]  UintegralTsProdOutMax=[]  UngainTsProdOutMin=[]  UngainTsProdOutMax=[]  IntegratorContinuousStateAttributes=''  IntegratorStateMustResolveToSignalObject=off  IntegratorRTWStateStorageClass=Auto  FilterContinuousStateAttributes=''  FilterStateMustResolveToSignalObject=off  FilterRTWStateStorageClass=Auto  ParallelPVariant=InternalParameters  IdealPVariant=Disabled  IVariant=InternalParameters  DVariant=InternalParameters  IntegratorVariant=Continuous  SatVariant=Disabled  AWVariant=Passthrough  PCopyVariant=Disabled  TRVariant=Disabled  FdbkBlocksVariant=Forward  IdealPFdbkVariant=Disabled  SatFdbkVariant=Disabled  DerivativeFilterVariant=ContFilter  NVariant=InternalParameters  NCopyVariant=Disabled  FilterICVariant=InternalICsFilter  IntegratorICVariant=InternalICs  ExternalResetVariant=Disabled  TRSumVariant=Passthrough  SumFdbkVariant=Disabled  SumVariant=Sum_PID  TsampFilterVariant=InternalTs  TsampNgainVariant=Passthrough  TsampIntegralVariant=Passthrough  ExternalSaturationOutDataTypeStr=Inherit: Same as second input  aMode=0
  Saturation1 : Saturate  UpperLimit=max_torque  LowerLimit=-max_torque
  Square : Math  Operator=square
  Square1 : Math  Operator=square
  Sum : Sum  Inputs=|++
  Sum1 : Sum  Inputs=+|+
  Sum2 : Sum  Inputs=|-+
  InputL : Outport
  Machine_State : Outport  Port=2
  wires:
  Mux/1 -> InputL/1
  Constant2/1 -> Machine_State/1
  Saturation1/1 -> Mux/1
  Data Store Read/1 -> Sum/1  "impact angle"
  PID Controller2/1 -> Saturation1/1
  Constant1/1 -> Mux/2
  Bus Selector1/2 -> Square1/1  "<Yd>"
  Square/1 -> Sum1/1
  Bus Selector1/1 -> Square/1  "<Xd>"
  measBody/1 -> Bus Selector1/1
  Square1/1 -> Sum1/2
  Gain/1 -> Sum/2  "desired speed"
  Sum/1 -> PID Controller2/1
  Constant/1 -> Sum2/2
  Sum1/1 -> Sum2/1
  Sum2/1 -> Gain/1

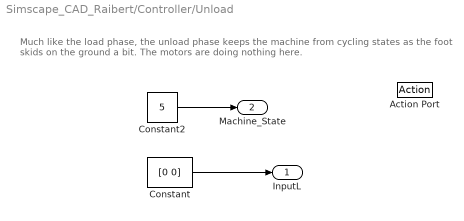
== system Simscape_CAD_Raibert/Controller/Unload ==
  note: Much like the load phase, the unload phase keeps the machine from cycling states as the foot skids on the ground a bit. The motors are doing nothing here.
  Action Port : ActionPort
      settings: CopyFcn=Stateflow.SLINSF.SimulinkMan.removeBlockPreDeleteFcn  PreDeleteFcn=Stateflow.SLINSF.SimulinkMan.unsafePredeleteFcn
  Constant : Constant  Value=[0 0]  VectorParams1D=off
  Constant2 : Constant  Value=5
  InputL : Outport
  Machine_State : Outport  Port=2
  wires:
  Constant/1 -> InputL/1
  Constant2/1 -> Machine_State/1
